simulink model "speedgoat_v2_minimal"  (R2021a)
settings: Solver=FixedStepDiscrete  StartTime=0.0  StopTime=inf  FixedStep=0.002  RelTol=1e-3
model workspace (MAT data in the model file):
  SGV2_SPEED_COMMAND_60FF = 0
  SGV2_SPEED_LIMIT_607F = 1000
libraries: slrealtimeethercatlib x10
settings Model: SimulationMode=external  Creator=Zemin  LastModifiedBy=Zemin
settings SolverCC: ConcurrentTasks=on  PositivePriorityOrder=on
settings OptimizationCC: BlockReduction=off  OptimizeBlockIOStorage=off
settings HardwareCC: ProdBitPerLong=64  ProdLongLongMode=on  ProdHWDeviceType=Intel->x86-64 (Linux 64)
settings RTWCC: Description=Simulink Real-Time  SystemTargetFile=slrealtime.tlc  TemplateMakefile=slrealtime_default_tmf  Toolchain=Simulink Real-Time Toolchain  BuildConfiguration=Faster Runs  CodeExecutionProfiling=on  TargetLang=C++

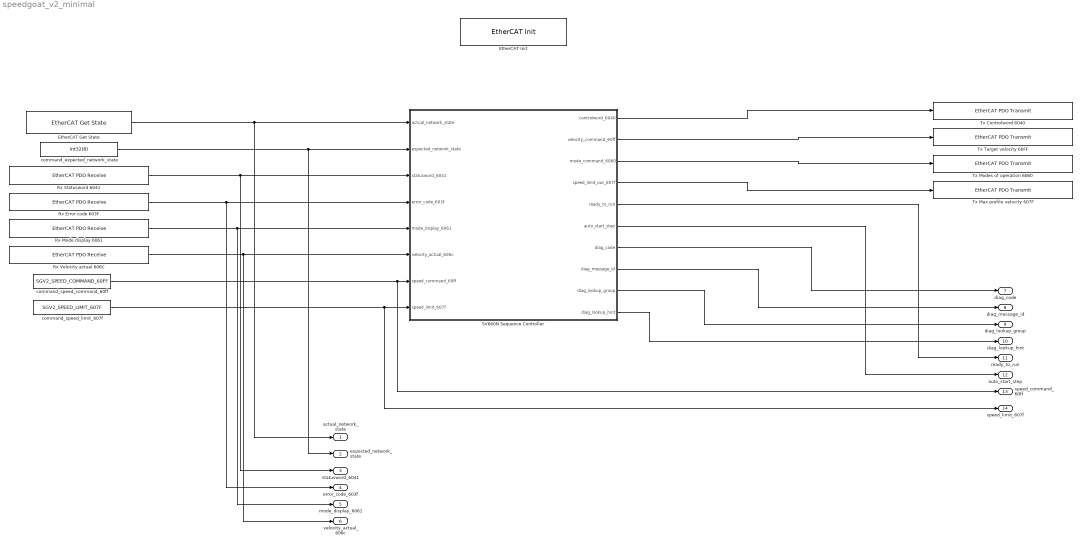
== system speedgoat_v2_minimal ==
  EtherCAT Get State : slrealtimeethercatlib/EtherCAT Get State  device_id=0  sample_time=0.002
      settings: SourceProductBaseCode=XP
  EtherCAT Init : slrealtimeethercatlib/EtherCAT Init  Priority=0  config_file=D:\Temporary_file\speedgoat_v2.0.0\matlab\config\ethercat\eni\ENI2.xml  device_id=0  pci_bus=0  pci_slot=0  pci_function=0  portnum=1  initstate=2  dctuning=0  enaDebug=0  enaDC=on  errLink=off  masterDbg=off  stateChgDbg=off  baseClock=off  masterCfg=off  logFile='c:\dbglog.txt'  sample_time=0.002000  DCMode=2
      settings: SourceProductBaseCode=XP
  Rx Error code 603F : slrealtimeethercatlib/EtherCAT PDO Receive  Priority=2  sig_name=Drive 1 (InoSV660N).Inputs.Error code  sig_offset=568  sig_type=uint16  type_size=16  sig_dim=1  device_id=0  sample_time=0.002000
      settings: SourceProductBaseCode=XP
  Rx Mode display 6061 : slrealtimeethercatlib/EtherCAT PDO Receive  Priority=2  sig_name=Drive 1 (InoSV660N).Inputs.Modes of operation display  sig_offset=648  sig_type=int8  type_size=8  sig_dim=1  device_id=0  sample_time=0.002000
      settings: SourceProductBaseCode=XP
  Rx Statusword 6041 : slrealtimeethercatlib/EtherCAT PDO Receive  Priority=2  sig_name=Drive 1 (InoSV660N).Inputs.Statusword  sig_offset=584  sig_type=uint16  type_size=16  sig_dim=1  device_id=0  sample_time=0.002000
      settings: SourceProductBaseCode=XP
  Rx Velocity actual 606C : slrealtimeethercatlib/EtherCAT PDO Receive  Priority=2  sig_name=Drive 1 (InoSV660N).Inputs.Velocity actual value  sig_offset=768  sig_type=int32  type_size=32  sig_dim=1  device_id=0  sample_time=0.002000
      settings: SourceProductBaseCode=XP
  SV660N Sequence Controller : Subsystem
  Tx Controlword 6040 : slrealtimeethercatlib/EtherCAT PDO Transmit  Priority=3  sig_name=Drive 1 (InoSV660N).Outputs.Controlword  sig_offset=568  sig_type=uint16  type_size=16  sig_dim=1  device_id=0  sample_time=0.002
      settings: SourceProductBaseCode=XP
  Tx Max profile velocity 607F : slrealtimeethercatlib/EtherCAT PDO Transmit  Priority=3  sig_name=Drive 1 (InoSV660N).Outputs.Max profile velocity  sig_offset=688  sig_type=uint32  type_size=32  sig_dim=1  device_id=0  sample_time=0.002
      settings: SourceProductBaseCode=XP
  Tx Modes of operation 6060 : slrealtimeethercatlib/EtherCAT PDO Transmit  Priority=3  sig_name=Drive 1 (InoSV660N).Outputs.Modes of operation  sig_offset=664  sig_type=int8  type_size=8  sig_dim=1  device_id=0  sample_time=0.002
      settings: SourceProductBaseCode=XP
  Tx Target velocity 60FF : slrealtimeethercatlib/EtherCAT PDO Transmit  Priority=3  sig_name=Drive 1 (InoSV660N).Outputs.Target velocity  sig_offset=616  sig_type=int32  type_size=32  sig_dim=1  device_id=0  sample_time=0.002
      settings: SourceProductBaseCode=XP
  command_expected_network_state : Constant  Value=int32(8)
  command_speed_command_60ff : Constant  Value=SGV2_SPEED_COMMAND_60FF
  command_speed_limit_607f : Constant  Value=SGV2_SPEED_LIMIT_607F
  actual_network_state : Outport
  expected_network_state : Outport  Port=2
  statusword_6041 : Outport  Port=3
  error_code_603f : Outport  Port=4
  mode_display_6061 : Outport  Port=5
  velocity_actual_606c : Outport  Port=6
  diag_code : Outport  Port=7
  diag_message_id : Outport  Port=8
  diag_lookup_group : Outport  Port=9
  diag_lookup_hint : Outport  Port=10
  ready_to_run : Outport  Port=11
  auto_start_step : Outport  Port=12
  speed_command_60ff : Outport  Port=13
  speed_limit_607f : Outport  Port=14
  wires:
  EtherCAT Get State/1 -> SV660N Sequence Controller/1(actual_network_state), actual_network_state/1
  Rx Statusword 6041/1 -> SV660N Sequence Controller/3(statusword_6041), statusword_6041/1
  Rx Error code 603F/1 -> SV660N Sequence Controller/4(error_code_603f), error_code_603f/1
  Rx Mode display 6061/1 -> SV660N Sequence Controller/5(mode_display_6061), mode_display_6061/1
  Rx Velocity actual 606C/1 -> SV660N Sequence Controller/6(velocity_actual_606c), velocity_actual_606c/1
  SV660N Sequence Controller/1(controlword_6040) -> Tx Controlword 6040/1
  SV660N Sequence Controller/2(velocity_command_60ff) -> Tx Target velocity 60FF/1
  SV660N Sequence Controller/3(mode_command_6060) -> Tx Modes of operation 6060/1
  SV660N Sequence Controller/4(speed_limit_out_607f) -> Tx Max profile velocity 607F/1
  command_expected_network_state/1 -> SV660N Sequence Controller/2(expected_network_state), expected_network_state/1
  command_speed_command_60ff/1 -> SV660N Sequence Controller/7(speed_command_60ff), speed_command_60ff/1
  command_speed_limit_607f/1 -> SV660N Sequence Controller/8(speed_limit_607f), speed_limit_607f/1
  SV660N Sequence Controller/7(diag_code) -> diag_code/1
  SV660N Sequence Controller/8(diag_message_id) -> diag_message_id/1
  SV660N Sequence Controller/9(diag_lookup_group) -> diag_lookup_group/1
  SV660N Sequence Controller/10(diag_lookup_hint) -> diag_lookup_hint/1
  SV660N Sequence Controller/5(ready_to_run) -> ready_to_run/1
  SV660N Sequence Controller/6(auto_start_step) -> auto_start_step/1

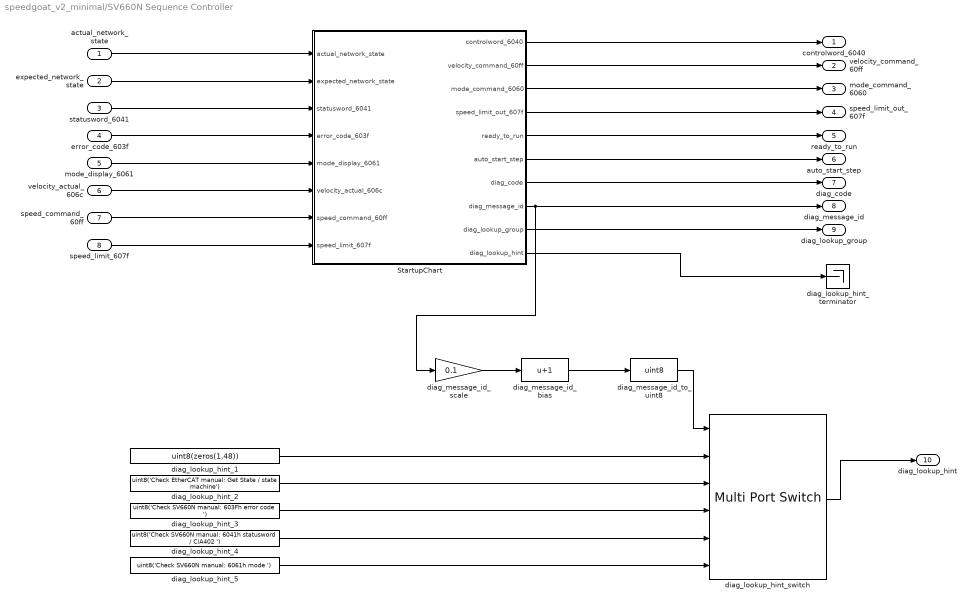
== system speedgoat_v2_minimal/SV660N Sequence Controller ==
  actual_network_state : Inport
  expected_network_state : Inport  Port=2
  statusword_6041 : Inport  Port=3
  error_code_603f : Inport  Port=4
  mode_display_6061 : Inport  Port=5
  velocity_actual_606c : Inport  Port=6
  speed_command_60ff : Inport  Port=7
  speed_limit_607f : Inport  Port=8
  StartupChart : Stateflow chart  TreatAsAtomicUnit=on
  diag_lookup_hint_1 : Constant  Value=uint8(zeros(1,48))  OutDataTypeStr=uint8
  diag_lookup_hint_2 : Constant  Value=uint8('Check EtherCAT manual: Get State / state machine')  OutDataTypeStr=uint8
  diag_lookup_hint_3 : Constant  Value="uint8('Check SV660N manual: 603Fh error code           ')"  OutDataTypeStr=uint8
  diag_lookup_hint_4 : Constant  Value="uint8('Check SV660N manual: 6041h statusword / CiA402  ')"  OutDataTypeStr=uint8
  diag_lookup_hint_5 : Constant  Value="uint8('Check SV660N manual: 6061h mode                 ')"  OutDataTypeStr=uint8
  diag_lookup_hint_switch : MultiPortSwitch  Inputs=5
  diag_lookup_hint_terminator : Terminator
  diag_message_id_bias : Bias  Bias=1
  diag_message_id_scale : Gain  Gain=0.1
  diag_message_id_to_uint8 : DataTypeConversion  OutDataTypeStr=uint8
  controlword_6040 : Outport
  velocity_command_60ff : Outport  Port=2
  mode_command_6060 : Outport  Port=3
  speed_limit_out_607f : Outport  Port=4
  ready_to_run : Outport  Port=5
  auto_start_step : Outport  Port=6
  diag_code : Outport  Port=7
  diag_message_id : Outport  Port=8
  diag_lookup_group : Outport  Port=9
  diag_lookup_hint : Outport  Port=10
  wires:
  actual_network_state/1 -> StartupChart/1(actual_network_state)
  expected_network_state/1 -> StartupChart/2(expected_network_state)
  statusword_6041/1 -> StartupChart/3(statusword_6041)
  error_code_603f/1 -> StartupChart/4(error_code_603f)
  mode_display_6061/1 -> StartupChart/5(mode_display_6061)
  velocity_actual_606c/1 -> StartupChart/6(velocity_actual_606c)
  speed_command_60ff/1 -> StartupChart/7(speed_command_60ff)
  speed_limit_607f/1 -> StartupChart/8(speed_limit_607f)
  StartupChart/1(controlword_6040) -> controlword_6040/1
  StartupChart/2(velocity_command_60ff) -> velocity_command_60ff/1
  StartupChart/3(mode_command_6060) -> mode_command_6060/1
  StartupChart/4(speed_limit_out_607f) -> speed_limit_out_607f/1
  StartupChart/5(ready_to_run) -> ready_to_run/1
  StartupChart/6(auto_start_step) -> auto_start_step/1
  StartupChart/7(diag_code) -> diag_code/1
  StartupChart/8(diag_message_id) -> diag_message_id_scale/1, diag_message_id/1
  StartupChart/9(diag_lookup_group) -> diag_lookup_group/1
  StartupChart/10(diag_lookup_hint) -> diag_lookup_hint_terminator/1
  diag_message_id_scale/1 -> diag_message_id_bias/1
  diag_message_id_bias/1 -> diag_message_id_to_uint8/1
  diag_message_id_to_uint8/1 -> diag_lookup_hint_switch/1
  diag_lookup_hint_1/1 -> diag_lookup_hint_switch/2
  diag_lookup_hint_2/1 -> diag_lookup_hint_switch/3
  diag_lookup_hint_3/1 -> diag_lookup_hint_switch/4
  diag_lookup_hint_4/1 -> diag_lookup_hint_switch/5
  diag_lookup_hint_5/1 -> diag_lookup_hint_switch/6
  diag_lookup_hint_switch/1 -> diag_lookup_hint/1

== stateflow chart speedgoat_v2_minimal/SV660N Sequence Controller/StartupChart ==
  state Run
    during:
    controlword_6040 = sgv2.controlword('disable_voltage');
    velocity_command_60ff = int32(0);
    mode_command_6060 = int8(9);
    speed_limit_out_607f = speed_limit_607f;
    ready_to_run = uint8(0);
    auto_start_step = sgv2.internal.autoStartStepIds().WAIT_BUS_OP;
    diag_code = sgv2.internal.diagCodes().NONE;
    diag_message_id = sgv2.internal.diagMessageIds().NONE;
    diag_lookup_group = sgv2.internal.diagLookupGroups().NONE;
    diag_lookup_hint = uint8(zeros(1, 48));
    if int32(actual_network_state) ~= int32(expected_network_state)
    auto_start_step = sgv2.internal.autoStartStepIds().WAIT_BUS_OP;
    diag_code = sgv2.internal.diagCodes().BUS_NOT_OP;
    diag_message_id = sgv2.internal.diagMessageIds().CHECK_ETHERCAT_STATE;
    diag_lookup_group = sgv2.internal.diagLookupGroups().ETHERCAT;
    elseif uint16(error_code_603f) ~= uint16(0)
    auto_start_step = sgv2.internal.autoStartStepIds().WAIT_DRIVE_CLEAR;
    diag_code = sgv2.internal.diagCodes().DRIVE_ERROR;
    diag_message_id = sgv2.internal.diagMessageIds().CHECK_603F;
    diag_lookup_group = sgv2.internal.diagLookupGroups().ERROR_CODE_603F;
    elseif sgv2.statusState(statusword_6041) >= sgv2.internal.faultStatusSentinel()
    auto_start_step = sgv2.internal.autoStartStepIds().WAIT_DRIVE_CLEAR;
    diag_code = sgv2.internal.diagCodes().DRIVE_FAULT;
    diag_message_id = sgv2.internal.diagMessageIds().CHECK_6041;
    diag_lookup_group = sgv2.internal.diagLookupGroups().STATUSWORD_6041;
    elseif sgv2.statusState(statusword_6041) == uint8(1)
    auto_start_step = sgv2.internal.autoStartStepIds().AUTO_POWER_ON;
    controlword_6040 = sgv2.controlword('shutdown');
    elseif sgv2.statusState(statusword_6041) == uint8(2)
    auto_start_step = sgv2.internal.autoStartStepIds().AUTO_ENABLE;
    controlword_6040 = sgv2.controlword('switch_on');
    elseif sgv2.statusState(statusword_6041) == uint8(3)
    auto_start_step = sgv2.internal.autoStartStepIds().AUTO_ENABLE;
    controlword_6040 = sgv2.controlword('enable_operation');
    elseif sgv2.statusState(statusword_6041) == uint8(4) && int8(mode_display_6061) ~= int8(9)
    auto_start_step = sgv2.internal.autoStartStepIds().AUTO_ENABLE;
    controlword_6040 = sgv2.controlword('enable_operation');
    diag_code = sgv2.internal.diagCodes().MODE_MISMATCH;
    diag_message_id = sgv2.internal.diagMessageIds().CHECK_6061;
    diag_lookup_group = sgv2.internal.diagLookupGroups().MODE_DISPLAY_6061;
    elseif sgv2.statusState(statusword_6041) == uint8(4)
    auto_start_step = sgv2.internal.autoStartStepIds().READY_TO_RUN;
    controlword_6040 = sgv2.controlword('enable_operation');
    velocity_command_60ff = speed_command_60ff;
    ready_to_run = uint8(1);
    else
    auto_start_step = sgv2.internal.autoStartStepIds().WAIT_DRIVE_CLEAR;
    diag_code = sgv2.internal.diagCodes().WAITING_ENABLE;
    diag_message_id = sgv2.internal.diagMessageIds().CHECK_6041;
    diag_lookup_group = sgv2.internal.diagLookupGroups().STATUSWORD_6041;
    end
    diag_lookup_hint = uint8(zeros(1, 48));
    if diag_message_id == sgv2.internal.diagMessageIds().NONE
    diag_lookup_hint = uint8(zeros(1, 48));
    end
  (default) -> Run
  data: actual_network_state input int32 size=1; expected_network_state input int32 size=1; statusword_6041 input uint16 size=1; error_code_603f input uint16 size=1; mode_display_6061 input int8 size=1; velocity_actual_606c input int32 size=1; speed_command_60ff input int32 size=1; speed_limit_607f input uint32 size=1; controlword_6040 output uint16 size=1; velocity_command_60ff output int32 size=1; mode_command_6060 output int8 size=1; speed_limit_out_607f output uint32 size=1; ready_to_run output uint8 size=1; auto_start_step output uint8 size=1; diag_code output uint8 size=1; diag_message_id output uint8 size=1; diag_lookup_group output uint8 size=1; diag_lookup_hint output uint8 size=[1 48] =uint8(zeros(1,48))
